simulink model "rocket_task_definition_process_modell"  (R2019a)
settings: Solver=VariableStepAuto  StartTime=0.0  StopTime=10.0  RelTol=1e-3
values from neighbouring files (symbols this model uses):
  ss_A = [0 1 0 0; 0 0 a23 0; 0 0 0 1; 0 0 a43 0]    [V2_A4_ZR_separ_nonlin_Aufgabenstellung.m]    (also in rocket.m = [0 1 0 0; 0 0 a1 0; 0 0 0 1; 0 0 a2 0]; rocket_task_definition.m; torpedo_tom_ole__09_12_19.m = [-1/T_RM 0 0; K_IS/T_NOMOTO -1/T_NOMOTO 0; 0 1 0])
  ss_B = [0; b2; 0; b4]    [V2_A4_ZR_separ_nonlin_Aufgabenstellung.m]    (also in rocket.m = [0; b1; 0; b2]; rocket_task_definition.m; torpedo_tom_ole__09_12_19.m = [K_RM/T_RM; 0; 0])
  ss_C = [1 0 0 0; 0 1 0 0; 0 0 1 0; 0 0 0 1]    [V2_A4_ZR_separ_nonlin_Aufgabenstellung.m]    (also in rocket.m; rocket_task_definition.m; torpedo_tom_ole__09_12_19.m = [0 0 1])
  ss_C1 = [1 0 0 0]    [V2_A4_ZR_separ_nonlin_Aufgabenstellung.m]    (also in rocket.m; rocket_task_definition.m)
settings Model: Creator=Jan  LastModifiedBy=Jan

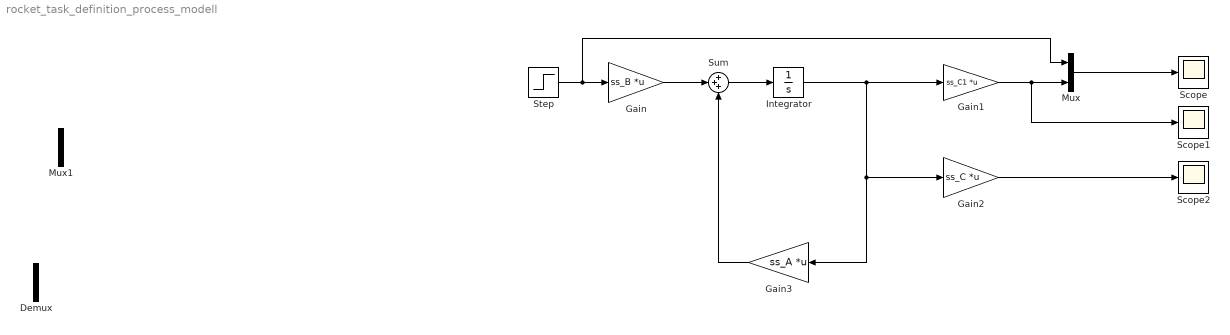
== system rocket_task_definition_process_modell ==
  Demux : Demux  Outputs=2
  Gain : Gain  Gain=ss_B  Multiplication=Matrix(K*u)
  Gain1 : Gain  Gain=ss_C1  Multiplication=Matrix(K*u)
  Gain2 : Gain  Gain=ss_C  Multiplication=Matrix(K*u)
  Gain3 : Gain  Gain=ss_A  Multiplication=Matrix(K*u)
  Integrator : Integrator
  Mux : Mux  Inputs=2
  Mux1 : Mux  Inputs=2
  Scope : Scope
  Scope1 : Scope
  Scope2 : Scope
  Step : Step  SampleTime=0
  Sum : Sum  Inputs=+++
  wires:
  Step/1 -> Gain/1, Mux/1
  Gain/1 -> Sum/2
  Sum/1 -> Integrator/1
  Integrator/1 -> Gain1/1, Gain2/1, Gain3/1
  Gain1/1 -> Mux/2, Scope1/1
  Mux/1 -> Scope/1
  Gain2/1 -> Scope2/1
  Gain3/1 -> Sum/3
